simulink model "closedloop"  (R2014a)
settings: Solver=ode45  StartTime=0.0  StopTime=tf  RelTol=1e-3
values from neighbouring files (symbols this model uses):
  beta_drag = 0.324    [driver.m]    (also in run_closedloop.m)
  k = 4774.65    [driver.m]    (also in run_closedloop.m)
  m = 1500    [driver.m]    (also in run_closedloop.m)
  tau_1 = 50    [driver.m]    (also in run_closedloop.m)
  tau_2 = 5    [driver.m]    (also in run_closedloop.m)
  u_eq = (beta_drag/k)*((v_star)^2)    (= 0.0610725393484)    [run_closedloop.m]
  x1_init = 27    [run_closedloop.m]
  x2_init = 262    [run_closedloop.m]
  x3_init = 0    [run_closedloop.m]
  y_eq = v_star    (= 30)    [run_closedloop.m]
undefined symbols (not defined in the file or in its folder): den_con, num_con
settings Model: Creator=sriramkswamy  LastModifiedBy=sriramkswamy
settings DataIOCC: SaveFormat=StructureWithTime  SaveState=on

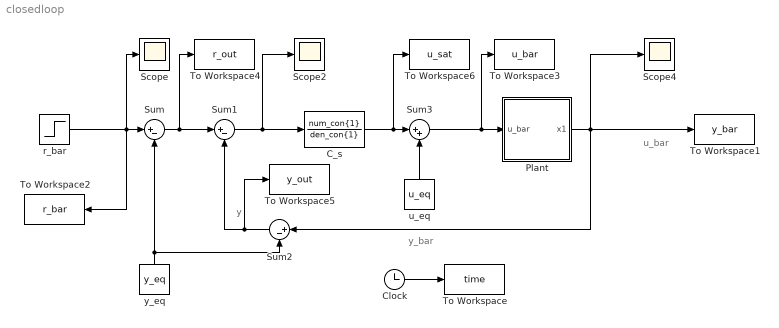
== system closedloop ==
  note: y_bar
  note: y
  note: u_bar
  C_s : TransferFcn  Numerator=num_con{1}  Denominator=den_con{1}
  Clock : Clock
  Plant : Subsystem
  Scope : Scope
  Scope2 : Scope
      settings: SaveName=ScopeData2
  Scope4 : Scope
      settings: SaveName=ScopeData4
  Sum : Sum  Inputs=|+-
  Sum1 : Sum  Inputs=|+-
  Sum2 : Sum  Inputs=|+-
  Sum3 : Sum  Inputs=|++
  To Workspace : ToWorkspace  VariableName=time  SaveFormat=Timeseries  SampleTime=-1
  To Workspace1 : ToWorkspace  VariableName=y_bar  SaveFormat=Timeseries  SampleTime=-1
  To Workspace2 : ToWorkspace  VariableName=r_bar  SaveFormat=Timeseries  SampleTime=-1
  To Workspace3 : ToWorkspace  VariableName=u_bar  SaveFormat=Timeseries  SampleTime=-1
  To Workspace4 : ToWorkspace  VariableName=r_out  SaveFormat=Timeseries  SampleTime=-1
  To Workspace5 : ToWorkspace  VariableName=y_out  SaveFormat=Timeseries  SampleTime=-1
  To Workspace6 : ToWorkspace  VariableName=u_sat  SaveFormat=Timeseries  SampleTime=-1
  r_bar : Step  Time=300  Before=31.111  After=33.333  SampleTime=0
  u_eq : Constant  Value=u_eq
  y_eq : Constant  Value=y_eq
  wires:
  r_bar/1 -> Scope/1, To Workspace2/1, Sum/1
  Sum/1 -> To Workspace4/1, Sum1/1
  Sum2/1 -> Sum1/2, To Workspace5/1
  y_eq/1 -> Sum/2, Sum2/2
  u_eq/1 -> Sum3/2
  C_s/1 -> To Workspace6/1, Sum3/1
  Clock/1 -> To Workspace/1
  Plant/1(x1) -> To Workspace1/1, Scope4/1, Sum2/1
  Sum3/1 -> Plant/1(u_bar), To Workspace3/1
  Sum1/1 -> C_s/1, Scope2/1

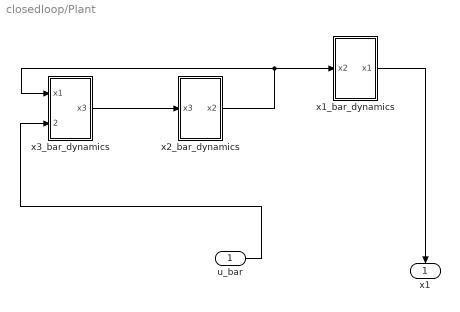
== system closedloop/Plant ==
  u_bar : Inport
  "x1_bar_dynamics " : Subsystem
  x2_bar_dynamics : Subsystem
  x3_bar_dynamics : Subsystem
  x1 : Outport
  wires:
  x2_bar_dynamics/1(x2) -> x3_bar_dynamics/1(x1), "x1_bar_dynamics "/1(x2)
  x3_bar_dynamics/1(x3) -> x2_bar_dynamics/1(x3)
  u_bar/1 -> x3_bar_dynamics/2(u_bar)
  "x1_bar_dynamics "/1(x1) -> x1/1

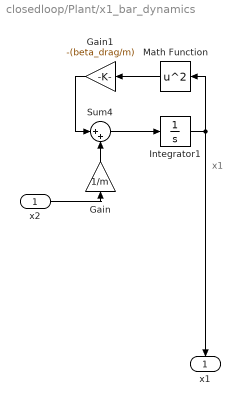
== system closedloop/Plant/x1_bar_dynamics  ==
  note: x1
  x2 : Inport
  Gain : Gain  Gain=1/m
  Gain1 : Gain  Gain=-(beta_drag/m)
  Integrator1 : Integrator  InitialCondition=x1_init
  Math Function : Math  Operator=square  SaturateOnIntegerOverflow=on
  Sum4 : Sum  Inputs=|++
  x1 : Outport
  wires:
  Math Function/1 -> Gain1/1
  Sum4/1 -> Integrator1/1
  Gain/1 -> Sum4/2
  x2/1 -> Gain/1
  Gain1/1 -> Sum4/1
  Integrator1/1 -> x1/1, Math Function/1

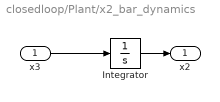
== system closedloop/Plant/x2_bar_dynamics ==
  x3 : Inport
  Integrator : Integrator  InitialCondition=x2_init
  x2 : Outport
  wires:
  x3/1 -> Integrator/1
  Integrator/1 -> x2/1

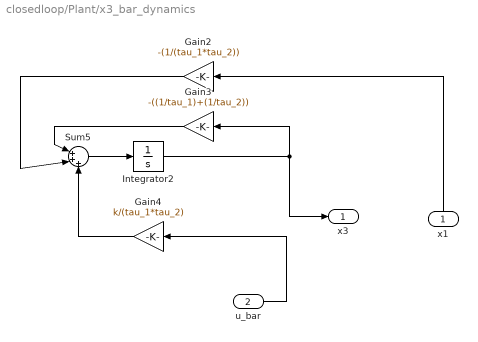
== system closedloop/Plant/x3_bar_dynamics ==
  x1 : Inport
  u_bar : Inport  Port=2
  Gain2 : Gain  Gain=-(1/(tau_1*tau_2))
  Gain3 : Gain  Gain=-((1/tau_1)+(1/tau_2))
  Gain4 : Gain  Gain=k/(tau_1*tau_2)
  Integrator2 : Integrator  InitialCondition=x3_init
  Sum5 : Sum  Inputs=|+++
  x3 : Outport
  wires:
  x1/1 -> Gain2/1
  Gain2/1 -> Sum5/2
  Gain4/1 -> Sum5/3
  Gain3/1 -> Sum5/1
  Integrator2/1 -> x3/1, Gain3/1
  Sum5/1 -> Integrator2/1
  u_bar/1 -> Gain4/1
